simulink model "benign"  (R2017a)
settings: Solver=FixedStepDiscrete  StartTime=0.0  StopTime=100  FixedStep=1  RelTol=1e-3
model workspace (MAT data in the model file):
  ContractValidatorBlocksMap = containers.Map
  ContractValidatorBlocksMap.serialization.keys = {'benign/con_uas/validator', 'benign/contract/validator'}
  ContractValidatorBlocksMap.serialization.values{1}.block = 'benign/con_uas/validator'
  ContractValidatorBlocksMap.serialization.values{1}.assumePorts = 0
  ContractValidatorBlocksMap.serialization.values{1}.guaranteePorts = 8
  ContractValidatorBlocksMap.serialization.values{1}.modeBlocksPorts = 0
  ContractValidatorBlocksMap.serialization.values{1}.portHandles.Inport = [5488.14013672 5489.13989258 5490.13989258 5491.13989258 5492.13989258 5493.13989258 5494.13989258 5495.13989258]
  ContractValidatorBlocksMap.serialization.values{1}.portHandles.Outport = 5496.13989258
  ContractValidatorBlocksMap.serialization.values{1}.portHandles.Enable = []
  ContractValidatorBlocksMap.serialization.values{1}.portHandles.Trigger = []
  ContractValidatorBlocksMap.serialization.values{1}.portHandles.State = []
  ContractValidatorBlocksMap.serialization.values{1}.portHandles.LConn = []
  ContractValidatorBlocksMap.serialization.values{1}.portHandles.RConn = []
  ContractValidatorBlocksMap.serialization.values{1}.portHandles.Ifaction = []
  ContractValidatorBlocksMap.serialization.values{1}.portHandles.Reset = []
  ContractValidatorBlocksMap.serialization.values{1}.portConnectivity(1).Type = '1'
  ContractValidatorBlocksMap.serialization.values{1}.portConnectivity(1).Position = [390 -490]
  ContractValidatorBlocksMap.serialization.values{1}.portConnectivity(1).SrcBlock = 98.0086669922
  ContractValidatorBlocksMap.serialization.values{1}.portConnectivity(1).SrcPort = 0
  ContractValidatorBlocksMap.serialization.values{1}.portConnectivity(1).DstBlock = []
  ContractValidatorBlocksMap.serialization.values{1}.portConnectivity(1).DstPort = []
  ContractValidatorBlocksMap.serialization.values{1}.portConnectivity(2).Type = '2'
  ContractValidatorBlocksMap.serialization.values{1}.portConnectivity(2).Position = [390 -275]
  ContractValidatorBlocksMap.serialization.values{1}.portConnectivity(2).SrcBlock = 126.00793457
  ContractValidatorBlocksMap.serialization.values{1}.portConnectivity(2).SrcPort = 0
  ContractValidatorBlocksMap.serialization.values{1}.portConnectivity(2).DstBlock = []
  ContractValidatorBlocksMap.serialization.values{1}.portConnectivity(2).DstPort = []
  ContractValidatorBlocksMap.serialization.values{1}.portConnectivity(3).Type = '3'
  ContractValidatorBlocksMap.serialization.values{1}.portConnectivity(3).Position = [390 -60]
  ContractValidatorBlocksMap.serialization.values{1}.portConnectivity(3).SrcBlock = 154.008300781
  ContractValidatorBlocksMap.serialization.values{1}.portConnectivity(3).SrcPort = 0
  ContractValidatorBlocksMap.serialization.values{1}.portConnectivity(3).DstBlock = []
  ContractValidatorBlocksMap.serialization.values{1}.portConnectivity(3).DstPort = []
  ContractValidatorBlocksMap.serialization.values{1}.portConnectivity(4).Type = '4'
  ContractValidatorBlocksMap.serialization.values{1}.portConnectivity(4).Position = [390 155]
  ContractValidatorBlocksMap.serialization.values{1}.portConnectivity(4).SrcBlock = 184.007324219
  ContractValidatorBlocksMap.serialization.values{1}.portConnectivity(4).SrcPort = 0
  ContractValidatorBlocksMap.serialization.values{1}.portConnectivity(4).DstBlock = []
  ContractValidatorBlocksMap.serialization.values{1}.portConnectivity(4).DstPort = []
  ContractValidatorBlocksMap.serialization.values{1}.portConnectivity(5).Type = '5'
  ContractValidatorBlocksMap.serialization.values{1}.portConnectivity(5).Position = [390 370]
  ContractValidatorBlocksMap.serialization.values{1}.portConnectivity(5).SrcBlock = 214.006591797
  ContractValidatorBlocksMap.serialization.values{1}.portConnectivity(5).SrcPort = 0
  ContractValidatorBlocksMap.serialization.values{1}.portConnectivity(5).DstBlock = []
  ContractValidatorBlocksMap.serialization.values{1}.portConnectivity(5).DstPort = []
  ContractValidatorBlocksMap.serialization.values{1}.portConnectivity(6).Type = '6'
  ContractValidatorBlocksMap.serialization.values{1}.portConnectivity(6).Position = [390 585]
  ContractValidatorBlocksMap.serialization.values{1}.portConnectivity(6).SrcBlock = 254.006347656
  ContractValidatorBlocksMap.serialization.values{1}.portConnectivity(6).SrcPort = 0
  ContractValidatorBlocksMap.serialization.values{1}.portConnectivity(6).DstBlock = []
  ContractValidatorBlocksMap.serialization.values{1}.portConnectivity(6).DstPort = []
  ContractValidatorBlocksMap.serialization.values{1}.portConnectivity(7).Type = '7'
  ContractValidatorBlocksMap.serialization.values{1}.portConnectivity(7).Position = [390 800]
  ContractValidatorBlocksMap.serialization.values{1}.portConnectivity(7).SrcBlock = 294.005859375
  ContractValidatorBlocksMap.serialization.values{1}.portConnectivity(7).SrcPort = 0
  ContractValidatorBlocksMap.serialization.values{1}.portConnectivity(7).DstBlock = []
  ContractValidatorBlocksMap.serialization.values{1}.portConnectivity(7).DstPort = []
  ContractValidatorBlocksMap.serialization.values{1}.portConnectivity(8).Type = '8'
  ContractValidatorBlocksMap.serialization.values{1}.portConnectivity(8).Position = [390 1015]
  ContractValidatorBlocksMap.serialization.values{1}.portConnectivity(8).SrcBlock = 334.007080078
  ContractValidatorBlocksMap.serialization.values{1}.portConnectivity(8).SrcPort = 0
  ContractValidatorBlocksMap.serialization.values{1}.portConnectivity(8).DstBlock = []
  ContractValidatorBlocksMap.serialization.values{1}.portConnectivity(8).DstPort = []
  ContractValidatorBlocksMap.serialization.values{1}.portConnectivity(9).Type = '1'
  ContractValidatorBlocksMap.serialization.values{1}.portConnectivity(9).Position = [615 265]
  ContractValidatorBlocksMap.serialization.values{1}.portConnectivity(9).SrcBlock = []
  ContractValidatorBlocksMap.serialization.values{1}.portConnectivity(9).SrcPort = []
  ContractValidatorBlocksMap.serialization.values{1}.portConnectivity(9).DstBlock = 376.00793457
  ContractValidatorBlocksMap.serialization.values{1}.portConnectivity(9).DstPort = 0
  ContractValidatorBlocksMap.serialization.values{2}.block = 'benign/contract/validator'
  ContractValidatorBlocksMap.serialization.values{2}.assumePorts = 1
  ContractValidatorBlocksMap.serialization.values{2}.guaranteePorts = 1
  ContractValidatorBlocksMap.serialization.values{2}.modeBlocksPorts = 3
  ContractValidatorBlocksMap.serialization.values{2}.portHandles.Inport = [15090.0004883 15091.0004883 14397.0036621 15089.0006104 14391.0037842]
  ContractValidatorBlocksMap.serialization.values{2}.portHandles.Outport = 5595.05529785
  ContractValidatorBlocksMap.serialization.values{2}.portHandles.Enable = []
  ContractValidatorBlocksMap.serialization.values{2}.portHandles.Trigger = []
  ContractValidatorBlocksMap.serialization.values{2}.portHandles.State = []
  ContractValidatorBlocksMap.serialization.values{2}.portHandles.LConn = []
  ContractValidatorBlocksMap.serialization.values{2}.portHandles.RConn = []
  ContractValidatorBlocksMap.serialization.values{2}.portHandles.Ifaction = []
  ContractValidatorBlocksMap.serialization.values{2}.portHandles.Reset = []
  ContractValidatorBlocksMap.serialization.values{2}.portConnectivity(1).Type = '1'
  ContractValidatorBlocksMap.serialization.values{2}.portConnectivity(1).Position = [365 -125]
  ContractValidatorBlocksMap.serialization.values{2}.portConnectivity(1).SrcBlock = 15175.0004883
  ContractValidatorBlocksMap.serialization.values{2}.portConnectivity(1).SrcPort = 0
  ContractValidatorBlocksMap.serialization.values{2}.portConnectivity(1).DstBlock = []
  ContractValidatorBlocksMap.serialization.values{2}.portConnectivity(1).DstPort = []
  ContractValidatorBlocksMap.serialization.values{2}.portConnectivity(2).Type = '2'
  ContractValidatorBlocksMap.serialization.values{2}.portConnectivity(2).Position = [365 -25]
  ContractValidatorBlocksMap.serialization.values{2}.portConnectivity(2).SrcBlock = 15178.0007324
  ContractValidatorBlocksMap.serialization.values{2}.portConnectivity(2).SrcPort = 0
  ContractValidatorBlocksMap.serialization.values{2}.portConnectivity(2).DstBlock = []
  ContractValidatorBlocksMap.serialization.values{2}.portConnectivity(2).DstPort = []
  ContractValidatorBlocksMap.serialization.values{2}.portConnectivity(3).Type = '3'
  ContractValidatorBlocksMap.serialization.values{2}.portConnectivity(3).Position = [365 75]
  ContractValidatorBlocksMap.serialization.values{2}.portConnectivity(3).SrcBlock = 15181.0007324
  ContractValidatorBlocksMap.serialization.values{2}.portConnectivity(3).SrcPort = 0
  ContractValidatorBlocksMap.serialization.values{2}.portConnectivity(3).DstBlock = []
  ContractValidatorBlocksMap.serialization.values{2}.portConnectivity(3).DstPort = []
  ContractValidatorBlocksMap.serialization.values{2}.portConnectivity(4).Type = '4'
  ContractValidatorBlocksMap.serialization.values{2}.portConnectivity(4).Position = [365 175]
  ContractValidatorBlocksMap.serialization.values{2}.portConnectivity(4).SrcBlock = 15204.0007324
  ContractValidatorBlocksMap.serialization.values{2}.portConnectivity(4).SrcPort = 0
  ContractValidatorBlocksMap.serialization.values{2}.portConnectivity(4).DstBlock = []
  ContractValidatorBlocksMap.serialization.values{2}.portConnectivity(4).DstPort = []
  ContractValidatorBlocksMap.serialization.values{2}.portConnectivity(5).Type = '5'
  ContractValidatorBlocksMap.serialization.values{2}.portConnectivity(5).Position = [365 275]
  ContractValidatorBlocksMap.serialization.values{2}.portConnectivity(5).SrcBlock = 15227.0007324
  ContractValidatorBlocksMap.serialization.values{2}.portConnectivity(5).SrcPort = 0
  ContractValidatorBlocksMap.serialization.values{2}.portConnectivity(5).DstBlock = []
  ContractValidatorBlocksMap.serialization.values{2}.portConnectivity(5).DstPort = []
  ContractValidatorBlocksMap.serialization.values{2}.portConnectivity(6).Type = '1'
  ContractValidatorBlocksMap.serialization.values{2}.portConnectivity(6).Position = [500 75]
  ContractValidatorBlocksMap.serialization.values{2}.portConnectivity(6).SrcBlock = []
  ContractValidatorBlocksMap.serialization.values{2}.portConnectivity(6).SrcPort = []
  ContractValidatorBlocksMap.serialization.values{2}.portConnectivity(6).DstBlock = 5588.05688477
  ContractValidatorBlocksMap.serialization.values{2}.portConnectivity(6).DstPort = 0
  ContractValidatorBlocksMap.serialization.uniformity = 0
  ContractValidatorBlocksMap.serialization.keyType = 'char'
  ContractValidatorBlocksMap.serialization.valueType = 'any'
undefined symbols (not defined in the file or in its folder): contractAfterSimulation, contractBeforeSimulation, saveValidatorParameters
undefined symbols (not defined in the file): ContractBlock, ContractGuaranteeBlock, ContractValidatorBlock
libraries: simulink x436, CoCoSimSpecification x31
(part 1 of 3)
settings Model: Creator=mudat  LastModifiedBy=mudat

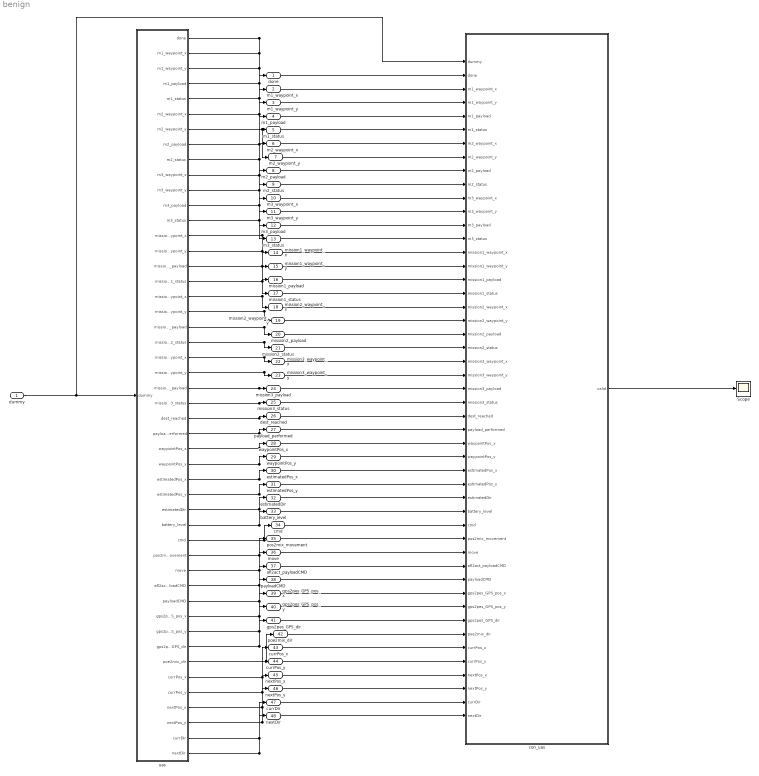
== system benign ==
  dummy : Inport  OutDataTypeStr=boolean
  Scope : Scope
  con_uas : Subsystem  mask(ContractBlock){ContractBlockType=ContractBlock}
      mask init:
      | set_param(gcb, 'LinkStatus', 'none');
      settings: CopyFcn=set_param(gcb, 'LinkStatus', 'none');
      mask DialogControl DescTextVar Prompt: Contract block
      mask Display:
      | text(0.5, 0.5, '{\bf\fontsize{20}Contract}', 'hor', 'center', 'texmode','on');
      | blocks = find_system(gcb, 'LookUnderMasks','all', 'SearchDepth',1,'BlockType','Inport');
      | for i = 1 : length(blocks)
      |     blockName = get_param(blocks(i), 'Name');
      |     [path, blockName] = fileparts(char(blockName));
      |     port_label('input', i, blockName);
      | end
      | 
      | blocks = find_system(gcb, 'LookUnderMasks','all', 'SearchDepth',1,'BlockType','Outport');
      | for i = 1 : length(blocks)
      |     blockName = get_param(blocks(i), 'Name');
      |     [path, blockName] = fileparts(char(blockName));
      |     port_label('output', i, blockName);
      | end
  uas : Subsystem
  done : Outport  OutDataTypeStr=boolean
  m1_waypoint_x : Outport  Port=2  OutDataTypeStr=int32
  m1_waypoint_y : Outport  Port=3  OutDataTypeStr=int32
  m1_payload : Outport  Port=4  OutDataTypeStr=int32
  m1_status : Outport  Port=5  OutDataTypeStr=int32
  m2_waypoint_x : Outport  Port=6  OutDataTypeStr=int32
  m2_waypoint_y : Outport  Port=7  OutDataTypeStr=int32
  m2_payload : Outport  Port=8  OutDataTypeStr=int32
  m2_status : Outport  Port=9  OutDataTypeStr=int32
  m3_waypoint_x : Outport  Port=10  OutDataTypeStr=int32
  m3_waypoint_y : Outport  Port=11  OutDataTypeStr=int32
  m3_payload : Outport  Port=12  OutDataTypeStr=int32
  m3_status : Outport  Port=13  OutDataTypeStr=int32
  mission1_waypoint_x : Outport  Port=14  OutDataTypeStr=int32
  mission1_waypoint_y : Outport  Port=15  OutDataTypeStr=int32
  mission1_payload : Outport  Port=16  OutDataTypeStr=int32
  mission1_status : Outport  Port=17  OutDataTypeStr=int32
  mission2_waypoint_x : Outport  Port=18  OutDataTypeStr=int32
  mission2_waypoint_y : Outport  Port=19  OutDataTypeStr=int32
  mission2_payload : Outport  Port=20  OutDataTypeStr=int32
  mission2_status : Outport  Port=21  OutDataTypeStr=int32
  mission3_waypoint_x : Outport  Port=22  OutDataTypeStr=int32
  mission3_waypoint_y : Outport  Port=23  OutDataTypeStr=int32
  mission3_payload : Outport  Port=24  OutDataTypeStr=int32
  mission3_status : Outport  Port=25  OutDataTypeStr=int32
  dest_reached : Outport  Port=26  OutDataTypeStr=boolean
  payload_performed : Outport  Port=27  OutDataTypeStr=boolean
  waypointPos_x : Outport  Port=28  OutDataTypeStr=int32
  waypointPos_y : Outport  Port=29  OutDataTypeStr=int32
  estimatedPos_x : Outport  Port=30  OutDataTypeStr=int32
  estimatedPos_y : Outport  Port=31  OutDataTypeStr=int32
  estimatedDir : Outport  Port=32  OutDataTypeStr=int32
  battery_level : Outport  Port=33  OutDataTypeStr=int32
  cmd : Outport  Port=34  OutDataTypeStr=int32
  pos2mix_movement : Outport  Port=35  OutDataTypeStr=int32
  move : Outport  Port=36  OutDataTypeStr=int32
  afl2act_payloadCMD : Outport  Port=37  OutDataTypeStr=int32
  payloadCMD : Outport  Port=38  OutDataTypeStr=int32
  gps2pes_GPS_pos_x : Outport  Port=39  OutDataTypeStr=int32
  gps2pes_GPS_pos_y : Outport  Port=40  OutDataTypeStr=int32
  gps2pes_GPS_dir : Outport  Port=41  OutDataTypeStr=int32
  poe2mix_dir : Outport  Port=42  OutDataTypeStr=int32
  currPos_x : Outport  Port=43  OutDataTypeStr=int32
  currPos_y : Outport  Port=44  OutDataTypeStr=int32
  nextPos_x : Outport  Port=45  OutDataTypeStr=int32
  nextPos_y : Outport  Port=46  OutDataTypeStr=int32
  currDir : Outport  Port=47  OutDataTypeStr=int32
  nextDir : Outport  Port=48  OutDataTypeStr=int32
  wires:
  dummy/1 -> con_uas/1(dummy), uas/1(dummy)
  uas/1(done) -> done/1, con_uas/2(done)
  uas/2(m1_waypoint_x) -> m1_waypoint_x/1, con_uas/3(m1_waypoint_x)
  uas/3(m1_waypoint_y) -> m1_waypoint_y/1, con_uas/4(m1_waypoint_y)
  uas/4(m1_payload) -> m1_payload/1, con_uas/5(m1_payload)
  uas/5(m1_status) -> m1_status/1, con_uas/6(m1_status)
  uas/6(m2_waypoint_x) -> m2_waypoint_x/1, con_uas/7(m2_waypoint_x)
  uas/7(m2_waypoint_y) -> m2_waypoint_y/1, con_uas/8(m2_waypoint_y)
  uas/8(m2_payload) -> m2_payload/1, con_uas/9(m2_payload)
  uas/9(m2_status) -> m2_status/1, con_uas/10(m2_status)
  uas/10(m3_waypoint_x) -> m3_waypoint_x/1, con_uas/11(m3_waypoint_x)
  uas/11(m3_waypoint_y) -> m3_waypoint_y/1, con_uas/12(m3_waypoint_y)
  uas/12(m3_payload) -> m3_payload/1, con_uas/13(m3_payload)
  uas/13(m3_status) -> m3_status/1, con_uas/14(m3_status)
  uas/14(mission1_waypoint_x) -> mission1_waypoint_x/1, con_uas/15(mission1_waypoint_x)
  uas/15(mission1_waypoint_y) -> mission1_waypoint_y/1, con_uas/16(mission1_waypoint_y)
  uas/16(mission1_payload) -> mission1_payload/1, con_uas/17(mission1_payload)
  uas/17(mission1_status) -> mission1_status/1, con_uas/18(mission1_status)
  uas/18(mission2_waypoint_x) -> mission2_waypoint_x/1, con_uas/19(mission2_waypoint_x)
  uas/19(mission2_waypoint_y) -> mission2_waypoint_y/1, con_uas/20(mission2_waypoint_y)
  uas/20(mission2_payload) -> mission2_payload/1, con_uas/21(mission2_payload)
  uas/21(mission2_status) -> mission2_status/1, con_uas/22(mission2_status)
  uas/22(mission3_waypoint_x) -> mission3_waypoint_x/1, con_uas/23(mission3_waypoint_x)
  uas/23(mission3_waypoint_y) -> mission3_waypoint_y/1, con_uas/24(mission3_waypoint_y)
  uas/24(mission3_payload) -> mission3_payload/1, con_uas/25(mission3_payload)
  uas/25(mission3_status) -> mission3_status/1, con_uas/26(mission3_status)
  uas/26(dest_reached) -> dest_reached/1, con_uas/27(dest_reached)
  uas/27(payload_performed) -> payload_performed/1, con_uas/28(payload_performed)
  uas/28(waypointPos_x) -> waypointPos_x/1, con_uas/29(waypointPos_x)
  uas/29(waypointPos_y) -> waypointPos_y/1, con_uas/30(waypointPos_y)
  uas/30(estimatedPos_x) -> estimatedPos_x/1, con_uas/31(estimatedPos_x)
  uas/31(estimatedPos_y) -> estimatedPos_y/1, con_uas/32(estimatedPos_y)
  uas/32(estimatedDir) -> estimatedDir/1, con_uas/33(estimatedDir)
  uas/33(battery_level) -> battery_level/1, con_uas/34(battery_level)
  uas/34(cmd) -> cmd/1, con_uas/35(cmd)
  uas/35(pos2mix_movement) -> pos2mix_movement/1, con_uas/36(pos2mix_movement)
  uas/36(move) -> move/1, con_uas/37(move)
  uas/37(afl2act_payloadCMD) -> afl2act_payloadCMD/1, con_uas/38(afl2act_payloadCMD)
  uas/38(payloadCMD) -> payloadCMD/1, con_uas/39(payloadCMD)
  uas/39(gps2pes_GPS_pos_x) -> gps2pes_GPS_pos_x/1, con_uas/40(gps2pes_GPS_pos_x)
  uas/40(gps2pes_GPS_pos_y) -> gps2pes_GPS_pos_y/1, con_uas/41(gps2pes_GPS_pos_y)
  uas/41(gps2pes_GPS_dir) -> gps2pes_GPS_dir/1, con_uas/42(gps2pes_GPS_dir)
  uas/42(poe2mix_dir) -> poe2mix_dir/1, con_uas/43(poe2mix_dir)
  uas/43(currPos_x) -> currPos_x/1, con_uas/44(currPos_x)
  uas/44(currPos_y) -> currPos_y/1, con_uas/45(currPos_y)
  uas/45(nextPos_x) -> nextPos_x/1, con_uas/46(nextPos_x)
  uas/46(nextPos_y) -> nextPos_y/1, con_uas/47(nextPos_y)
  uas/47(currDir) -> currDir/1, con_uas/48(currDir)
  uas/48(nextDir) -> nextDir/1, con_uas/49(nextDir)
  con_uas/1(valid) -> Scope/1

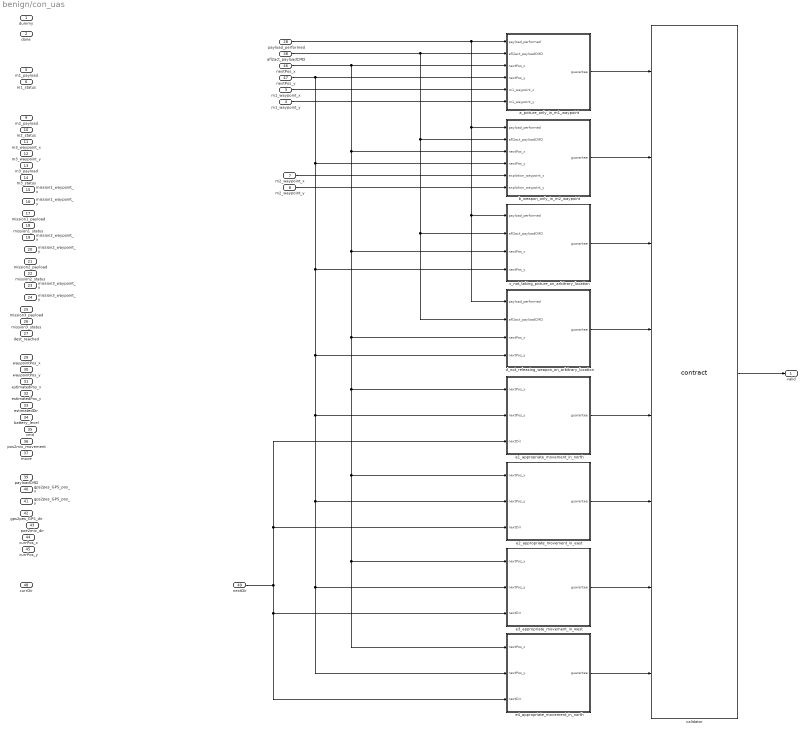
== system benign/con_uas ==
  dummy : Inport
  done : Inport  Port=2
  m1_waypoint_x : Inport  Port=3
  m1_waypoint_y : Inport  Port=4
  m1_payload : Inport  Port=5
  m1_status : Inport  Port=6
  m2_waypoint_x : Inport  Port=7
  m2_waypoint_y : Inport  Port=8
  m2_payload : Inport  Port=9
  m2_status : Inport  Port=10
  m3_waypoint_x : Inport  Port=11
  m3_waypoint_y : Inport  Port=12
  m3_payload : Inport  Port=13
  m3_status : Inport  Port=14
  mission1_waypoint_x : Inport  Port=15
  mission1_waypoint_y : Inport  Port=16
  mission1_payload : Inport  Port=17
  mission1_status : Inport  Port=18
  mission2_waypoint_x : Inport  Port=19
  mission2_waypoint_y : Inport  Port=20
  mission2_payload : Inport  Port=21
  mission2_status : Inport  Port=22
  mission3_waypoint_x : Inport  Port=23
  mission3_waypoint_y : Inport  Port=24
  mission3_payload : Inport  Port=25
  mission3_status : Inport  Port=26
  dest_reached : Inport  Port=27
  payload_performed : Inport  Port=28
  waypointPos_x : Inport  Port=29
  waypointPos_y : Inport  Port=30
  estimatedPos_x : Inport  Port=31
  estimatedPos_y : Inport  Port=32
  estimatedDir : Inport  Port=33
  battery_level : Inport  Port=34
  cmd : Inport  Port=35
  pos2mix_movement : Inport  Port=36
  move : Inport  Port=37
  afl2act_payloadCMD : Inport  Port=38
  payloadCMD : Inport  Port=39
  gps2pes_GPS_pos_x : Inport  Port=40
  gps2pes_GPS_pos_y : Inport  Port=41
  gps2pes_GPS_dir : Inport  Port=42
  poe2mix_dir : Inport  Port=43
  currPos_x : Inport  Port=44
  currPos_y : Inport  Port=45
  nextPos_x : Inport  Port=46
  nextPos_y : Inport  Port=47
  currDir : Inport  Port=48
  nextDir : Inport  Port=49
  a_picture_only_in_m1_waypoint : Subsystem  mask(ContractGuaranteeBlock){ContractBlockType=ContractGuaranteeBlock}
      mask init:
      | set_param(gcb, 'LinkStatus', 'none');
      mask DialogControl DescTextVar Prompt: Guarantee block
  b_weapon_only_in_m2_waypoint : Subsystem  mask(ContractGuaranteeBlock){ContractBlockType=ContractGuaranteeBlock}
      mask init:
      | set_param(gcb, 'LinkStatus', 'none');
      mask DialogControl DescTextVar Prompt: Guarantee block
  c_not_taking_picture_on_arbitrary_location : Subsystem  mask(ContractGuaranteeBlock){ContractBlockType=ContractGuaranteeBlock}
      mask init:
      | set_param(gcb, 'LinkStatus', 'none');
      mask DialogControl DescTextVar Prompt: Guarantee block
  d_not_releasing_weapon_on_arbitrary_location : Subsystem  mask(ContractGuaranteeBlock){ContractBlockType=ContractGuaranteeBlock}
      mask init:
      | set_param(gcb, 'LinkStatus', 'none');
      mask DialogControl DescTextVar Prompt: Guarantee block
  e1_appropriate_movement_in_north : Subsystem  mask(ContractGuaranteeBlock){ContractBlockType=ContractGuaranteeBlock}
      mask init:
      | set_param(gcb, 'LinkStatus', 'none');
      mask DialogControl DescTextVar Prompt: Guarantee block
  e2_appropriate_movement_in_east : Subsystem  mask(ContractGuaranteeBlock){ContractBlockType=ContractGuaranteeBlock}
      mask init:
      | set_param(gcb, 'LinkStatus', 'none');
      mask DialogControl DescTextVar Prompt: Guarantee block
  e3_appropriate_movement_in_west : Subsystem  mask(ContractGuaranteeBlock){ContractBlockType=ContractGuaranteeBlock}
      mask init:
      | set_param(gcb, 'LinkStatus', 'none');
      mask DialogControl DescTextVar Prompt: Guarantee block
  e4_appropriate_movement_in_north : Subsystem  mask(ContractGuaranteeBlock){ContractBlockType=ContractGuaranteeBlock}
      mask init:
      | set_param(gcb, 'LinkStatus', 'none');
      mask DialogControl DescTextVar Prompt: Guarantee block
  validator : M-S-Function  LoadFcn=saveValidatorParameters(gcb);  InitFcn=contractBeforeSimulation();  StopFcn=contractAfterSimulation();  FunctionName=contract  mask(ContractValidatorBlock){assumePorts=0, guaranteePorts=8, modePorts=0, ContractBlockType=ContractValidatorBlock, createInportsCheckbox=off}
      mask prompts: assumePorts "Assume ports     :"; guaranteePorts "Guarantee ports :"; modePorts "Mode ports        :"; createInportsCheckbox "Create inports and connect them automatically"
      mask init:
      | set_param(gcb,'LinkStatus','none');
      | contract_callback('inputs_callback',gcb);
      mask DialogControl DescTextVar Prompt: The validator block implements the following logic: <br> <br> <b>Sofar</b>(assume<sub>1</sub> <b>&#8743;</b> assume<sub>2</sub> <b>&#8743;</b> ... assume<sub>k</sub>) <b>&rarr;</b> (guarantee<sub>1</sub> <b>&#8743;</b> guarantee<sub>2</sub> <b>&#8743;</b> ... guarantee<sub>m</sub> <b>&#8743;</b>  mode<sub>1</sub> <b>&#8743;</b> mode<sub>2</sub> <b>&#8743;</b> ... <b>&#8743;</b> mode<sub>n</sub> )<br> where mode<sub>i</sub> = require<sub>i</sub> <b>&rarr;</b> ensure<sub>i</sub>
      mask Display:
      | color('black');
      | port_label('input',1,'guarantee');
      | port_label('input',2,'guarantee');
      | port_label('input',3,'guarantee');
      | port_label('input',4,'guarantee');
      | port_label('input',5,'guarantee');
      | port_label('input',6,'guarantee');
      | port_label('input',7,'guarantee');
      | port_label('input',8,'guarantee');
      | port_label('output',1,'valid');
  valid : Outport
  wires:
  validator/1 -> valid/1
  m1_waypoint_x/1 -> a_picture_only_in_m1_waypoint/5(m1_waypoint_x)
  m1_waypoint_y/1 -> a_picture_only_in_m1_waypoint/6(m1_waypoint_y)
  m2_waypoint_x/1 -> b_weapon_only_in_m2_waypoint/5(explotion_waypoint_x)
  m2_waypoint_y/1 -> b_weapon_only_in_m2_waypoint/6(explotion_waypoint_y)
  payload_performed/1 -> d_not_releasing_weapon_on_arbitrary_location/1(payload_performed), c_not_taking_picture_on_arbitrary_location/1(payload_performed), b_weapon_only_in_m2_waypoint/1(payload_performed), a_picture_only_in_m1_waypoint/1(payload_performed)
  afl2act_payloadCMD/1 -> d_not_releasing_weapon_on_arbitrary_location/2(afl2act_payloadCMD), c_not_taking_picture_on_arbitrary_location/2(afl2act_payloadCMD), b_weapon_only_in_m2_waypoint/2(afl2act_payloadCMD), a_picture_only_in_m1_waypoint/2(afl2act_payloadCMD)
  nextDir/1 -> e3_appropriate_movement_in_west/3(nextDir), e4_appropriate_movement_in_north/3(nextDir), e2_appropriate_movement_in_east/3(nextDir), e1_appropriate_movement_in_north/3(nextDir)
  a_picture_only_in_m1_waypoint/1(guarantee) -> validator/1
  b_weapon_only_in_m2_waypoint/1(guarantee) -> validator/2
  c_not_taking_picture_on_arbitrary_location/1(guarantee) -> validator/3
  d_not_releasing_weapon_on_arbitrary_location/1(guarantee) -> validator/4
  e1_appropriate_movement_in_north/1(guarantee) -> validator/5
  e2_appropriate_movement_in_east/1(guarantee) -> validator/6
  e3_appropriate_movement_in_west/1(guarantee) -> validator/7
  nextPos_x/1 -> e4_appropriate_movement_in_north/1(nextPos_x), e3_appropriate_movement_in_west/1(nextPos_x), e2_appropriate_movement_in_east/1(nextPos_x), e1_appropriate_movement_in_north/1(nextPos_x), d_not_releasing_weapon_on_arbitrary_location/3(nextPos_x), c_not_taking_picture_on_arbitrary_location/3(nextPos_x), b_weapon_only_in_m2_waypoint/3(nextPos_x), a_picture_only_in_m1_waypoint/3(nextPos_x)
  nextPos_y/1 -> e4_appropriate_movement_in_north/2(nextPos_y), e3_appropriate_movement_in_west/2(nextPos_y), e2_appropriate_movement_in_east/2(nextPos_y), e1_appropriate_movement_in_north/2(nextPos_y), d_not_releasing_weapon_on_arbitrary_location/4(nextPos_y), c_not_taking_picture_on_arbitrary_location/4(nextPos_y), b_weapon_only_in_m2_waypoint/4(nextPos_y), a_picture_only_in_m1_waypoint/4(nextPos_y)
  e4_appropriate_movement_in_north/1(guarantee) -> validator/8

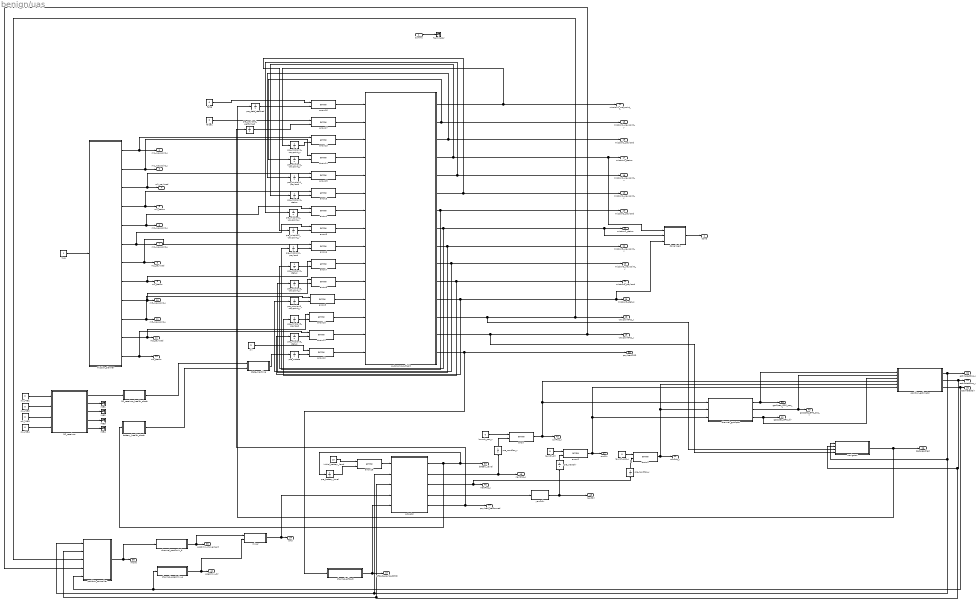
== system benign/uas ==
  dummy : Inport  OutDataTypeStr=boolean
  MIE{1..4} (4 alike) : Terminator
  RC_receiver : Subsystem
  RC_receiver_health_check : Subsystem
  Terminator : Terminator
  actuator : Subsystem
  arrow{,1..18} (19 alike) : CoCoSimSpecification/arrow  LustreOperatorBlock=ArrowOperator
      settings: SourceProductName=CoCoSim Specification
  autonomous_flight : Subsystem
  battery_health_check : Subsystem
  channel_afl2act : Subsystem
  channel_gps2pes : Subsystem
  channel_poe2mix_a : Subsystem
  channel_poe2mix_b : Subsystem
  done logic : Subsystem
  false : Constant  Value=0  OutDataTypeStr=boolean
  false1 : Constant  Value=0  OutDataTypeStr=boolean
  initial_battery_level : Constant  Value=15  OutDataTypeStr=int32
  launch_dir : Constant  Value=0  OutDataTypeStr=int32
  launch_pos_x : Constant  Value=0  OutDataTypeStr=int32
  launch_pos_y : Constant  Value=0  OutDataTypeStr=int32
  mission_planner : Subsystem
  mixer : Subsystem
  navigator : Subsystem
  position_controller : Subsystem
  position_estimator : Subsystem
  pre_battery_level : UnitDelay  SampleTime=-1
  pre_dest_reached : UnitDelay  SampleTime=-1
  pre_mission1_payload : UnitDelay  SampleTime=-1
  pre_mission1_status : UnitDelay  SampleTime=-1
  pre_mission1_waypoint_x : UnitDelay  SampleTime=-1
  pre_mission1_waypoint_y : UnitDelay  SampleTime=-1
  pre_mission2_payload : UnitDelay  SampleTime=-1
  pre_mission2_status : UnitDelay  SampleTime=-1
  pre_mission2_waypoint_x : UnitDelay  SampleTime=-1
  pre_mission2_waypoint_y : UnitDelay  SampleTime=-1
  pre_mission3_payload : UnitDelay  SampleTime=-1
  pre_mission3_status : UnitDelay  SampleTime=-1
  pre_mission3_waypoint_x : UnitDelay  SampleTime=-1
  pre_mission3_waypoint_y : UnitDelay  SampleTime=-1
  pre_mstate : UnitDelay  SampleTime=-1
  pre_nextDir : UnitDelay  SampleTime=-1
  pre_nextPos_x : UnitDelay  SampleTime=-1
  pre_nextPos_y : UnitDelay  SampleTime=-1
  pre_payload_performed : UnitDelay  SampleTime=-1
  rcv_MIE{1..4} (4 alike) : Constant  Value=0  OutDataTypeStr=int32
  six : Constant  Value=6  OutDataTypeStr=int32
  state_machine : Subsystem
  true : Constant  OutDataTypeStr=boolean
  yaw2dir : Subsystem
  done : Outport  OutDataTypeStr=boolean
  m1_waypoint_x : Outport  Port=2  OutDataTypeStr=int32
  m1_waypoint_y : Outport  Port=3  OutDataTypeStr=int32
  m1_payload : Outport  Port=4  OutDataTypeStr=int32
  m1_status : Outport  Port=5  OutDataTypeStr=int32
  m2_waypoint_x : Outport  Port=6  OutDataTypeStr=int32
  m2_waypoint_y : Outport  Port=7  OutDataTypeStr=int32
  m2_payload : Outport  Port=8  OutDataTypeStr=int32
  m2_status : Outport  Port=9  OutDataTypeStr=int32
  m3_waypoint_x : Outport  Port=10  OutDataTypeStr=int32
  m3_waypoint_y : Outport  Port=11  OutDataTypeStr=int32
  m3_payload : Outport  Port=12  OutDataTypeStr=int32
  m3_status : Outport  Port=13  OutDataTypeStr=int32
  mission1_waypoint_x : Outport  Port=14  OutDataTypeStr=int32
  mission1_waypoint_y : Outport  Port=15  OutDataTypeStr=int32
  mission1_payload : Outport  Port=16  OutDataTypeStr=int32
  mission1_status : Outport  Port=17  OutDataTypeStr=int32
  mission2_waypoint_x : Outport  Port=18  OutDataTypeStr=int32
  mission2_waypoint_y : Outport  Port=19  OutDataTypeStr=int32
  mission2_payload : Outport  Port=20  OutDataTypeStr=int32
  mission2_status : Outport  Port=21  OutDataTypeStr=int32
  mission3_waypoint_x : Outport  Port=22  OutDataTypeStr=int32
  mission3_waypoint_y : Outport  Port=23  OutDataTypeStr=int32
  mission3_payload : Outport  Port=24  OutDataTypeStr=int32
  mission3_status : Outport  Port=25  OutDataTypeStr=int32
  dest_reached : Outport  Port=26  OutDataTypeStr=boolean
  payload_performed : Outport  Port=27  OutDataTypeStr=boolean
  waypointPos_x : Outport  Port=28  OutDataTypeStr=int32
  waypointPos_y : Outport  Port=29  OutDataTypeStr=int32
  estimatedPos_x : Outport  Port=30  OutDataTypeStr=int32
  estimatedPos_y : Outport  Port=31  OutDataTypeStr=int32
  estimatedDir : Outport  Port=32  OutDataTypeStr=int32
  battery_level : Outport  Port=33  OutDataTypeStr=int32
  cmd : Outport  Port=34  OutDataTypeStr=int32
  pos2mix_movement : Outport  Port=35  OutDataTypeStr=int32
  move : Outport  Port=36  OutDataTypeStr=int32
  afl2act_payloadCMD : Outport  Port=37  OutDataTypeStr=int32
  payloadCMD : Outport  Port=38  OutDataTypeStr=int32
  gps2pes_GPS_pos_x : Outport  Port=39  OutDataTypeStr=int32
  gps2pes_GPS_pos_y : Outport  Port=40  OutDataTypeStr=int32
  gps2pes_GPS_dir : Outport  Port=41  OutDataTypeStr=int32
  poe2mix_dir : Outport  Port=42  OutDataTypeStr=int32
  currPos_x : Outport  Port=43  OutDataTypeStr=int32
  currPos_y : Outport  Port=44  OutDataTypeStr=int32
  nextPos_x : Outport  Port=45  OutDataTypeStr=int32
  nextPos_y : Outport  Port=46  OutDataTypeStr=int32
  currDir : Outport  Port=47  OutDataTypeStr=int32
  nextDir : Outport  Port=48  OutDataTypeStr=int32
  wires:
  true/1 -> mission_planner/1(dummy)
  mission_planner/1(m1_waypoint_x) -> arrow13/1, m1_waypoint_x/1
  mission_planner/2(m1_waypoint_y) -> arrow14/1, m1_waypoint_y/1
  mission_planner/3(m1_payload) -> arrow15/1, m1_payload/1
  mission_planner/4(m1_status) -> arrow3/1, m1_status/1
  mission_planner/5(m2_waypoint_x) -> arrow4/1, m2_waypoint_x/1
  mission_planner/6(m2_waypoint_y) -> m2_waypoint_y/1, arrow5/1
  mission_planner/7(m2_payload) -> arrow6/1, m2_payload/1
  mission_planner/8(m2_status) -> arrow7/1, m2_status/1
  mission_planner/9(m3_waypoint_x) -> arrow8/1, m3_waypoint_x/1
  mission_planner/10(m3_waypoint_y) -> arrow9/1, m3_waypoint_y/1
  mission_planner/11(m3_payload) -> arrow10/1, m3_payload/1
  mission_planner/12(m3_status) -> arrow11/1, m3_status/1
  launch_pos_x/1 -> arrow/1
  arrow/1 -> currPos_x/1, position_estimator/4(currPos_x), channel_gps2pes/1(currPos_x)
  launch_pos_y/1 -> arrow1/1
  arrow1/1 -> currPos_y/1, position_estimator/5(currPos_y), channel_gps2pes/2(currPos_y)
  actuator/1(new_battery_level) -> battery_health_check/1(battery_level), pre_battery_level/1, battery_level/1
  actuator/2(nextPos_x) -> nextPos_x/1, pre_nextPos_x/1
  actuator/3(nextPos_y) -> pre_nextPos_y/1, nextPos_y/1
  actuator/5(payload_performed) -> pre_payload_performed/1, payload_performed/1
  arrow2/1 -> channel_gps2pes/3(currDir), position_estimator/6(currDir), currDir/1
  launch_dir/1 -> arrow2/1
  actuator/4(yaw) -> yaw2dir/1(yaw)
  yaw2dir/1(dir) -> nextDir/1, pre_nextDir/1
  channel_gps2pes/1(gps2pes_GPS_pos_x) -> gps2pes_GPS_pos_x/1, position_estimator/1(gps2pes_GPS_pos_x)
  channel_gps2pes/2(gps2pes_GPS_pos_y) -> gps2pes_GPS_pos_y/1, position_estimator/2(gps2pes_GPS_pos_y)
  channel_gps2pes/3(gps2pes_GPS_dir) -> position_estimator/3(gps2pes_GPS_dir), gps2pes_GPS_dir/1
  position_estimator/1(estimatedPos_x) -> navigator/1(estimatedPos_x), position_controller/1(currentPos_x), actuator/2(currentPos_x), estimatedPos_x/1
  position_estimator/2(estimatedPos_y) -> position_controller/2(currentPos_y), actuator/3(currentPos_y), navigator/2(estimatedPos_y), estimatedPos_y/1
  position_estimator/3(estimatedDir) -> position_controller/5(currentDir), channel_poe2mix_a/1(in_dir), estimatedDir/1
  autonomous_flight/1(upd_mission1_waypoint_x) -> pre_mission1_waypoint_x/1, mission1_waypoint_x/1
  autonomous_flight/2(upd_mission1_waypoint_y) -> mission1_waypoint_y/1, pre_mission1_waypoint_y/1
  autonomous_flight/3(upd_mission1_payload) -> mission1_payload/1, pre_mission1_payload/1
  autonomous_flight/4(upd_mission1_status) -> done logic/1(mission1_status), mission1_status/1, pre_mission1_status/1
  autonomous_flight/5(upd_mission2_waypoint_x) -> mission2_waypoint_x/1, pre_mission2_waypoint_x/1
  autonomous_flight/6(upd_mission2_waypoint_y) -> pre_mission2_waypoint_y/1, mission2_waypoint_y/1
  autonomous_flight/7(upd_mission2_payload) -> mission2_payload/1, pre_mission2_payload/1
  autonomous_flight/8(upd_mission2_status) -> pre_mission2_status/1, done logic/2(mission2_status), mission2_status/1
  autonomous_flight/9(upd_mission3_waypoint_x) -> pre_mission3_waypoint_x/1, mission3_waypoint_x/1
  autonomous_flight/10(upd_mission3_waypoint_y) -> pre_mission3_waypoint_y/1, mission3_waypoint_y/1
  autonomous_flight/11(upd_mission3_payload) -> pre_mission3_payload/1, mission3_payload/1
  autonomous_flight/12(upd_mission3_status) -> pre_mission3_status/1, done logic/3(mission3_status), mission3_status/1
  autonomous_flight/13(waypointPos_x) -> navigator/3(waypointPos_x), position_controller/3(waypointPos_x), waypointPos_x/1
  autonomous_flight/14(waypointPos_y) -> position_controller/4(waypointPos_y), waypointPos_y/1, navigator/4(waypointPos_y)
  autonomous_flight/15(payloadCMD) -> channel_afl2act/1(in_payloadCMD), payloadCMD/1
  false/1 -> arrow16/1
  false1/1 -> arrow17/1
  navigator/1(dest_reached) -> pre_dest_reached/1, dest_reached/1
  arrow16/1 -> autonomous_flight/1(dest_reached)
  arrow17/1 -> autonomous_flight/2(payload_performed)
  pre_payload_performed/1 -> arrow17/2
  pre_dest_reached/1 -> arrow16/2
  pre_nextPos_y/1 -> arrow1/2
  pre_nextPos_x/1 -> arrow/2
  pre_nextDir/1 -> arrow2/2
  arrow13/1 -> autonomous_flight/3(mission1_waypoint_x)
  arrow12/1 -> autonomous_flight/15(mstate)
  arrow11/1 -> autonomous_flight/14(mission3_status)
  arrow10/1 -> autonomous_flight/13(mission3_payload)
  arrow9/1 -> autonomous_flight/12(mission3_waypoint_y)
  arrow8/1 -> autonomous_flight/11(mission3_waypoint_x)
  arrow7/1 -> autonomous_flight/10(mission2_status)
  arrow6/1 -> autonomous_flight/9(mission2_payload)
  arrow5/1 -> autonomous_flight/8(mission2_waypoint_y)
  arrow4/1 -> autonomous_flight/7(mission2_waypoint_x)
  arrow3/1 -> autonomous_flight/6(mission1_status)
  arrow15/1 -> autonomous_flight/5(mission1_payload)
  arrow14/1 -> autonomous_flight/4(mission1_waypoint_y)
  pre_mission1_waypoint_x/1 -> arrow13/2
  pre_mission1_waypoint_y/1 -> arrow14/2
  pre_mission1_status/1 -> arrow3/2
  pre_mission1_payload/1 -> arrow15/2
  pre_mission2_waypoint_x/1 -> arrow4/2
  pre_mission2_waypoint_y/1 -> arrow5/2
  pre_mission2_payload/1 -> arrow6/2
  pre_mission2_status/1 -> arrow7/2
  pre_mission3_waypoint_x/1 -> arrow8/2
  pre_mission3_waypoint_y/1 -> arrow9/2
  pre_mission3_payload/1 -> arrow10/2
  pre_mission3_status/1 -> arrow11/2
  pre_mstate/1 -> arrow12/2
  state_machine/1(mstate) -> pre_mstate/1
  six/1 -> arrow12/1
  done logic/1(done) -> done/1
  RC_receiver_health_check/1(ATE6) -> state_machine/1(ATE6)
  RC_receiver/1(normal) -> RC_receiver_health_check/1(normal)
  battery_health_check/1(ATE7) -> state_machine/2(ATE7)
  rcv_MIE1/1 -> RC_receiver/1(rcv_MIE1)
  rcv_MIE2/1 -> RC_receiver/2(rcv_MIE2)
  rcv_MIE3/1 -> RC_receiver/3(rcv_MIE3)
  rcv_MIE4/1 -> RC_receiver/4(rcv_MIE4)
  RC_receiver/2(MIE1) -> MIE1/1
  RC_receiver/5(MIE4) -> MIE4/1
  RC_receiver/4(MIE3) -> MIE3/1
  RC_receiver/3(MIE2) -> MIE2/1
  initial_battery_level/1 -> arrow18/1
  arrow18/1 -> actuator/1(battery_level)
  pre_battery_level/1 -> arrow18/2
  mixer/1(cmd) -> actuator/4(cmd), cmd/1
  channel_afl2act/1(out_payloadCMD) -> actuator/5(payloadCMD), afl2act_payloadCMD/1
  channel_poe2mix_a/1(out_dir) -> mixer/2(currentDir), poe2mix_dir/1
  channel_poe2mix_b/1(out_movement) -> mixer/1(move), pos2mix_movement/1
  position_controller/1(move) -> channel_poe2mix_b/1(in_movement), move/1
  dummy/1 -> Terminator/1

== system benign/con_uas/a_picture_only_in_m1_waypoint ==
  payload_performed : Inport  OutDataTypeStr=boolean
  afl2act_payloadCMD : Inport  Port=2  OutDataTypeStr=int32
  nextPos_x : Inport  Port=3  OutDataTypeStr=int32
  nextPos_y : Inport  Port=4  OutDataTypeStr=int32
  m1_waypoint_x : Inport  Port=5  OutDataTypeStr=int32
  m1_waypoint_y : Inport  Port=6  OutDataTypeStr=int32
  Compare To Constant : simulink/Logic and Bit Operations/Compare To Constant  relop===  const=0  OutDataTypeStr=boolean
  Logical Operator1 : Logic  Operator=NOT  IconShape=distinctive  AllPortsSameDT=off  OutDataTypeStr=boolean
  Relational Operator : RelationalOperator  Operator===  OutDataTypeStr=boolean  RndMeth=Simplest
  Relational Operator1 : RelationalOperator  Operator===  OutDataTypeStr=boolean  RndMeth=Simplest
  and : Logic  IconShape=distinctive  AllPortsSameDT=off  OutDataTypeStr=boolean
  and1 : Logic  IconShape=distinctive  AllPortsSameDT=off  OutDataTypeStr=boolean
  or : Logic  Operator=OR  IconShape=distinctive  AllPortsSameDT=off  OutDataTypeStr=boolean
  guarantee : Outport  OutDataTypeStr=boolean
  wires:
  payload_performed/1 -> and/1
  afl2act_payloadCMD/1 -> Compare To Constant/1
  Compare To Constant/1 -> and/2
  and/1 -> Logical Operator1/1
  Logical Operator1/1 -> or/1
  or/1 -> guarantee/1
  nextPos_x/1 -> Relational Operator/1
  m1_waypoint_x/1 -> Relational Operator/2
  nextPos_y/1 -> Relational Operator1/1
  m1_waypoint_y/1 -> Relational Operator1/2
  Relational Operator/1 -> and1/1
  Relational Operator1/1 -> and1/2
  and1/1 -> or/2

== system benign/con_uas/b_weapon_only_in_m2_waypoint ==
  payload_performed : Inport  OutDataTypeStr=boolean
  afl2act_payloadCMD : Inport  Port=2  OutDataTypeStr=int32
  nextPos_x : Inport  Port=3  OutDataTypeStr=int32
  nextPos_y : Inport  Port=4  OutDataTypeStr=int32
  explotion_waypoint_x : Inport  Port=5  OutDataTypeStr=int32
  explotion_waypoint_y : Inport  Port=6  OutDataTypeStr=int32
  Compare To Constant : simulink/Logic and Bit Operations/Compare To Constant  relop===  const=1  OutDataTypeStr=boolean
  Logical Operator1 : Logic  Operator=NOT  IconShape=distinctive  AllPortsSameDT=off  OutDataTypeStr=boolean
  Relational Operator : RelationalOperator  Operator===  OutDataTypeStr=boolean  RndMeth=Simplest
  Relational Operator1 : RelationalOperator  Operator===  OutDataTypeStr=boolean  RndMeth=Simplest
  and : Logic  IconShape=distinctive  AllPortsSameDT=off  OutDataTypeStr=boolean
  and1 : Logic  IconShape=distinctive  AllPortsSameDT=off  OutDataTypeStr=boolean
  or : Logic  Operator=OR  IconShape=distinctive  AllPortsSameDT=off  OutDataTypeStr=boolean
  guarantee : Outport  OutDataTypeStr=boolean
  wires:
  payload_performed/1 -> and/1
  afl2act_payloadCMD/1 -> Compare To Constant/1
  Compare To Constant/1 -> and/2
  and/1 -> Logical Operator1/1
  Logical Operator1/1 -> or/1
  or/1 -> guarantee/1
  nextPos_x/1 -> Relational Operator/1
  explotion_waypoint_x/1 -> Relational Operator/2
  nextPos_y/1 -> Relational Operator1/1
  explotion_waypoint_y/1 -> Relational Operator1/2
  Relational Operator/1 -> and1/1
  Relational Operator1/1 -> and1/2
  and1/1 -> or/2

== system benign/con_uas/c_not_taking_picture_on_arbitrary_location ==
  payload_performed : Inport  OutDataTypeStr=boolean
  afl2act_payloadCMD : Inport  Port=2  OutDataTypeStr=int32
  nextPos_x : Inport  Port=3  OutDataTypeStr=int32
  nextPos_y : Inport  Port=4  OutDataTypeStr=int32
  Compare To Constant : simulink/Logic and Bit Operations/Compare To Constant  relop===  const=0  OutDataTypeStr=boolean
  Constant : Constant  Value=0  OutDataTypeStr=int32
  Constant1 : Constant  OutDataTypeStr=int32
  Logical Operator1 : Logic  Operator=NOT  IconShape=distinctive  AllPortsSameDT=off  OutDataTypeStr=boolean
  Logical Operator2 : Logic  Operator=NOT  IconShape=distinctive  AllPortsSameDT=off  OutDataTypeStr=boolean
  Relational Operator : RelationalOperator  Operator===  OutDataTypeStr=boolean  RndMeth=Simplest
  Relational Operator1 : RelationalOperator  Operator===  OutDataTypeStr=boolean  RndMeth=Simplest
  and : Logic  IconShape=distinctive  AllPortsSameDT=off  OutDataTypeStr=boolean
  and1 : Logic  IconShape=distinctive  AllPortsSameDT=off  OutDataTypeStr=boolean
  or : Logic  Operator=OR  IconShape=distinctive  AllPortsSameDT=off  OutDataTypeStr=boolean
  guarantee : Outport  OutDataTypeStr=boolean
  wires:
  payload_performed/1 -> and/1
  afl2act_payloadCMD/1 -> Compare To Constant/1
  Compare To Constant/1 -> and/2
  and/1 -> Logical Operator1/1
  Logical Operator1/1 -> or/1
  or/1 -> guarantee/1
  nextPos_x/1 -> Relational Operator/1
  Constant/1 -> Relational Operator/2
  nextPos_y/1 -> Relational Operator1/1
  Constant1/1 -> Relational Operator1/2
  Relational Operator/1 -> and1/1
  Relational Operator1/1 -> and1/2
  and1/1 -> Logical Operator2/1
  Logical Operator2/1 -> or/2

== system benign/con_uas/d_not_releasing_weapon_on_arbitrary_location ==
  payload_performed : Inport  OutDataTypeStr=boolean
  afl2act_payloadCMD : Inport  Port=2  OutDataTypeStr=int32
  nextPos_x : Inport  Port=3  OutDataTypeStr=int32
  nextPos_y : Inport  Port=4  OutDataTypeStr=int32
  Compare To Constant : simulink/Logic and Bit Operations/Compare To Constant  relop===  const=1  OutDataTypeStr=boolean
  Constant : Constant  Value=3  OutDataTypeStr=int32
  Constant1 : Constant  OutDataTypeStr=int32
  Logical Operator1 : Logic  Operator=NOT  IconShape=distinctive  AllPortsSameDT=off  OutDataTypeStr=boolean
  Logical Operator2 : Logic  Operator=NOT  IconShape=distinctive  AllPortsSameDT=off  OutDataTypeStr=boolean
  Relational Operator : RelationalOperator  Operator===  OutDataTypeStr=boolean  RndMeth=Simplest
  Relational Operator1 : RelationalOperator  Operator===  OutDataTypeStr=boolean  RndMeth=Simplest
  and : Logic  IconShape=distinctive  AllPortsSameDT=off  OutDataTypeStr=boolean
  and1 : Logic  IconShape=distinctive  AllPortsSameDT=off  OutDataTypeStr=boolean
  or : Logic  Operator=OR  IconShape=distinctive  AllPortsSameDT=off  OutDataTypeStr=boolean
  guarantee : Outport  OutDataTypeStr=boolean
  wires:
  payload_performed/1 -> and/1
  afl2act_payloadCMD/1 -> Compare To Constant/1
  Compare To Constant/1 -> and/2
  and/1 -> Logical Operator1/1
  Logical Operator1/1 -> or/1
  or/1 -> guarantee/1
  nextPos_x/1 -> Relational Operator/1
  Constant/1 -> Relational Operator/2
  nextPos_y/1 -> Relational Operator1/1
  Constant1/1 -> Relational Operator1/2
  Relational Operator/1 -> and1/1
  Relational Operator1/1 -> and1/2
  and1/1 -> Logical Operator2/1
  Logical Operator2/1 -> or/2

== system benign/con_uas/e1_appropriate_movement_in_north ==
  nextPos_x : Inport  OutDataTypeStr=int32
  nextPos_y : Inport  Port=2  OutDataTypeStr=int32
  nextDir : Inport  Port=3  OutDataTypeStr=int32
  Add : Sum
  Logical Operator1 : Logic  Operator=NOT  IconShape=distinctive  AllPortsSameDT=off  OutDataTypeStr=boolean
  Relational Operator : RelationalOperator  Operator===  OutDataTypeStr=boolean  RndMeth=Simplest
  Relational Operator1 : RelationalOperator  Operator===  OutDataTypeStr=boolean  RndMeth=Simplest
  Relational Operator2 : RelationalOperator  Operator===  OutDataTypeStr=boolean  RndMeth=Simplest
  and : Logic  IconShape=distinctive  AllPortsSameDT=off  OutDataTypeStr=boolean
  arrow1 : CoCoSimSpecification/arrow  LustreOperatorBlock=ArrowOperator
      settings: SourceProductName=CoCoSim Specification
  one : Constant  OutDataTypeStr=int32
  or : Logic  Operator=OR  IconShape=distinctive  AllPortsSameDT=off  OutDataTypeStr=boolean
  pre_nextDir : UnitDelay  SampleTime=-1
  pre_nextPos_x : UnitDelay  SampleTime=-1
  pre_nextPos_y : UnitDelay  SampleTime=-1
  true : Constant  OutDataTypeStr=boolean
  zero : Constant  Value=0  OutDataTypeStr=int32
  guarantee : Outport  OutDataTypeStr=boolean
  wires:
  Relational Operator1/1 -> and/2
  Relational Operator/1 -> and/1
  nextPos_y/1 -> pre_nextPos_y/1, Relational Operator1/1
  nextPos_x/1 -> pre_nextPos_x/1, Relational Operator/1
  or/1 -> arrow1/2
  Logical Operator1/1 -> or/1
  true/1 -> arrow1/1
  pre_nextPos_x/1 -> Relational Operator/2
  pre_nextPos_y/1 -> Add/1
  Add/1 -> Relational Operator1/2
  one/1 -> Add/2
  nextDir/1 -> pre_nextDir/1
  pre_nextDir/1 -> Relational Operator2/1
  zero/1 -> Relational Operator2/2
  Relational Operator2/1 -> or/2
  and/1 -> Logical Operator1/1
  arrow1/1 -> guarantee/1

== system benign/con_uas/e2_appropriate_movement_in_east ==
  nextPos_x : Inport  OutDataTypeStr=int32
  nextPos_y : Inport  Port=2  OutDataTypeStr=int32
  nextDir : Inport  Port=3  OutDataTypeStr=int32
  Add1 : Sum
  Logical Operator1 : Logic  Operator=NOT  IconShape=distinctive  AllPortsSameDT=off  OutDataTypeStr=boolean
  Relational Operator : RelationalOperator  Operator===  OutDataTypeStr=boolean  RndMeth=Simplest
  Relational Operator1 : RelationalOperator  Operator===  OutDataTypeStr=boolean  RndMeth=Simplest
  Relational Operator2 : RelationalOperator  Operator===  OutDataTypeStr=boolean  RndMeth=Simplest
  and : Logic  IconShape=distinctive  AllPortsSameDT=off  OutDataTypeStr=boolean
  arrow1 : CoCoSimSpecification/arrow  LustreOperatorBlock=ArrowOperator
      settings: SourceProductName=CoCoSim Specification
  one1 : Constant  OutDataTypeStr=int32
  or : Logic  Operator=OR  IconShape=distinctive  AllPortsSameDT=off  OutDataTypeStr=boolean
  pre_nextDir : UnitDelay  SampleTime=-1
  pre_nextPos_x : UnitDelay  SampleTime=-1
  pre_nextPos_y : UnitDelay  SampleTime=-1
  true : Constant  OutDataTypeStr=boolean
  two : Constant  Value=2  OutDataTypeStr=int32
  guarantee : Outport  OutDataTypeStr=boolean
  wires:
  arrow1/1 -> guarantee/1
  and/1 -> Logical Operator1/1
  Relational Operator2/1 -> or/2
  two/1 -> Relational Operator2/2
  pre_nextDir/1 -> Relational Operator2/1
  nextDir/1 -> pre_nextDir/1
  pre_nextPos_y/1 -> Relational Operator1/2
  pre_nextPos_x/1 -> Add1/1
  true/1 -> arrow1/1
  Logical Operator1/1 -> or/1
  or/1 -> arrow1/2
  nextPos_x/1 -> Relational Operator/1, pre_nextPos_x/1
  nextPos_y/1 -> Relational Operator1/1, pre_nextPos_y/1
  Relational Operator/1 -> and/1
  Relational Operator1/1 -> and/2
  Add1/1 -> Relational Operator/2
  one1/1 -> Add1/2

== system benign/con_uas/e3_appropriate_movement_in_west ==
  nextPos_x : Inport  OutDataTypeStr=int32
  nextPos_y : Inport  Port=2  OutDataTypeStr=int32
  nextDir : Inport  Port=3  OutDataTypeStr=int32
  Add : Sum  Inputs=+-
  Logical Operator1 : Logic  Operator=NOT  IconShape=distinctive  AllPortsSameDT=off  OutDataTypeStr=boolean
  Relational Operator : RelationalOperator  Operator===  OutDataTypeStr=boolean  RndMeth=Simplest
  Relational Operator1 : RelationalOperator  Operator===  OutDataTypeStr=boolean  RndMeth=Simplest
  Relational Operator2 : RelationalOperator  Operator===  OutDataTypeStr=boolean  RndMeth=Simplest
  and : Logic  IconShape=distinctive  AllPortsSameDT=off  OutDataTypeStr=boolean
  arrow1 : CoCoSimSpecification/arrow  LustreOperatorBlock=ArrowOperator
      settings: SourceProductName=CoCoSim Specification
  one : Constant  OutDataTypeStr=int32
  or : Logic  Operator=OR  IconShape=distinctive  AllPortsSameDT=off  OutDataTypeStr=boolean
  pre_nextDir : UnitDelay  SampleTime=-1
  pre_nextPos_x : UnitDelay  SampleTime=-1
  pre_nextPos_y : UnitDelay  SampleTime=-1
  three : Constant  Value=3  OutDataTypeStr=int32
  true : Constant  OutDataTypeStr=boolean
  guarantee : Outport  OutDataTypeStr=boolean
  wires:
  Relational Operator1/1 -> and/2
  Relational Operator/1 -> and/1
  nextPos_y/1 -> pre_nextPos_y/1, Relational Operator1/1
  nextPos_x/1 -> pre_nextPos_x/1, Relational Operator/1
  or/1 -> arrow1/2
  Logical Operator1/1 -> or/1
  true/1 -> arrow1/1
  one/1 -> Add/2
  nextDir/1 -> pre_nextDir/1
  pre_nextDir/1 -> Relational Operator2/1
  three/1 -> Relational Operator2/2
  Relational Operator2/1 -> or/2
  and/1 -> Logical Operator1/1
  arrow1/1 -> guarantee/1
  Add/1 -> Relational Operator/2
  pre_nextPos_x/1 -> Add/1
  pre_nextPos_y/1 -> Relational Operator1/2

== system benign/con_uas/e4_appropriate_movement_in_north ==
  nextPos_x : Inport  OutDataTypeStr=int32
  nextPos_y : Inport  Port=2  OutDataTypeStr=int32
  nextDir : Inport  Port=3  OutDataTypeStr=int32
  Add : Sum  Inputs=+-
  Logical Operator1 : Logic  Operator=NOT  IconShape=distinctive  AllPortsSameDT=off  OutDataTypeStr=boolean
  Relational Operator : RelationalOperator  Operator===  OutDataTypeStr=boolean  RndMeth=Simplest
  Relational Operator1 : RelationalOperator  Operator===  OutDataTypeStr=boolean  RndMeth=Simplest
  Relational Operator2 : RelationalOperator  Operator===  OutDataTypeStr=boolean  RndMeth=Simplest
  and : Logic  IconShape=distinctive  AllPortsSameDT=off  OutDataTypeStr=boolean
  arrow1 : CoCoSimSpecification/arrow  LustreOperatorBlock=ArrowOperator
      settings: SourceProductName=CoCoSim Specification
  one : Constant  OutDataTypeStr=int32
  one1 : Constant  OutDataTypeStr=int32
  or : Logic  Operator=OR  IconShape=distinctive  AllPortsSameDT=off  OutDataTypeStr=boolean
  pre_nextDir : UnitDelay  SampleTime=-1
  pre_nextPos_x : UnitDelay  SampleTime=-1
  pre_nextPos_y : UnitDelay  SampleTime=-1
  true : Constant  OutDataTypeStr=boolean
  guarantee : Outport  OutDataTypeStr=boolean
  wires:
  arrow1/1 -> guarantee/1
  and/1 -> Logical Operator1/1
  Relational Operator2/1 -> or/2
  one1/1 -> Relational Operator2/2
  pre_nextDir/1 -> Relational Operator2/1
  nextDir/1 -> pre_nextDir/1
  one/1 -> Add/2
  Add/1 -> Relational Operator1/2
  pre_nextPos_y/1 -> Add/1
  pre_nextPos_x/1 -> Relational Operator/2
  true/1 -> arrow1/1
  Logical Operator1/1 -> or/1
  or/1 -> arrow1/2
  nextPos_x/1 -> Relational Operator/1, pre_nextPos_x/1
  nextPos_y/1 -> Relational Operator1/1, pre_nextPos_y/1
  Relational Operator/1 -> and/1
  Relational Operator1/1 -> and/2

== system benign/uas/RC_receiver ==
  rcv_MIE1 : Inport  OutDataTypeStr=int32
  rcv_MIE2 : Inport  Port=2  OutDataTypeStr=int32
  rcv_MIE3 : Inport  Port=3  OutDataTypeStr=int32
  rcv_MIE4 : Inport  Port=4  OutDataTypeStr=int32
  true : Constant  OutDataTypeStr=boolean
  normal : Outport  OutDataTypeStr=boolean
  MIE1 : Outport  Port=2  OutDataTypeStr=int32
  MIE2 : Outport  Port=3  OutDataTypeStr=int32
  MIE3 : Outport  Port=4  OutDataTypeStr=int32
  MIE4 : Outport  Port=5  OutDataTypeStr=int32
  wires:
  rcv_MIE4/1 -> MIE4/1
  rcv_MIE3/1 -> MIE3/1
  rcv_MIE2/1 -> MIE2/1
  rcv_MIE1/1 -> MIE1/1
  true/1 -> normal/1

== system benign/uas/RC_receiver_health_check ==
  normal : Inport  OutDataTypeStr=boolean
  Relational Operator : RelationalOperator  Operator=<=  OutDataTypeStr=boolean  RndMeth=Simplest
  Switch : Switch  Criteria=u2 > Threshold
  duration : Subsystem
  one : Constant  OutDataTypeStr=int32
  tolerance_level : Constant  OutDataTypeStr=int32
  zero : Constant  Value=0  OutDataTypeStr=int32
  ATE6 : Outport  OutDataTypeStr=int32
  wires:
  normal/1 -> duration/1(p)
  duration/1(r) -> Relational Operator/1
  tolerance_level/1 -> Relational Operator/2
  Relational Operator/1 -> Switch/2
  one/1 -> Switch/1
  zero/1 -> Switch/3
  Switch/1 -> ATE6/1

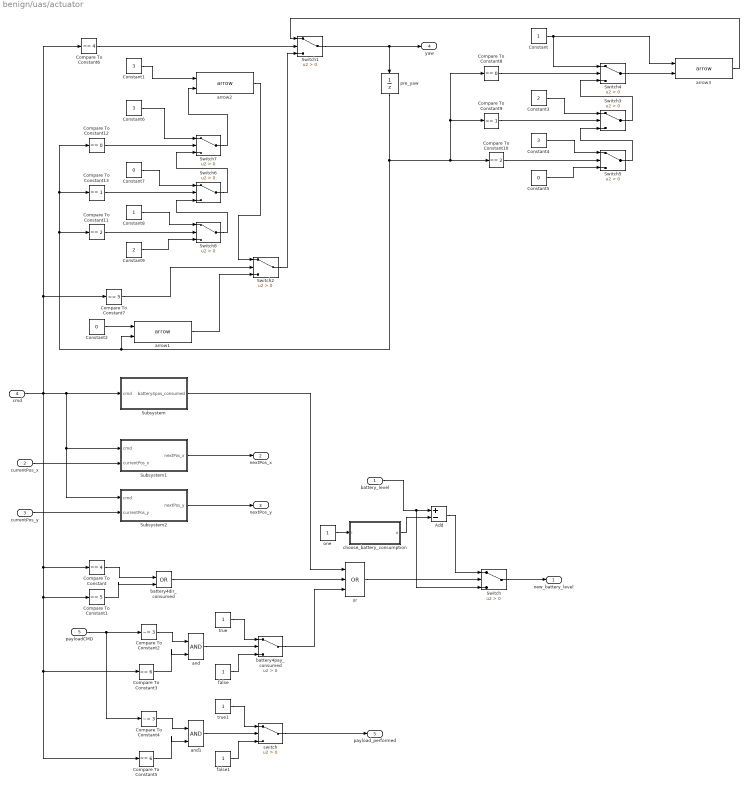
== system benign/uas/actuator ==
  battery_level : Inport  OutDataTypeStr=int32
  currentPos_x : Inport  Port=2  OutDataTypeStr=int32
  currentPos_y : Inport  Port=3  OutDataTypeStr=int32
  cmd : Inport  Port=4  OutDataTypeStr=int32
  payloadCMD : Inport  Port=5  OutDataTypeStr=int32
  Add : Sum  Inputs=+-
  Compare To Constant : simulink/Logic and Bit Operations/Compare To Constant  relop===  const=4  OutDataTypeStr=boolean
  Compare To Constant1 : simulink/Logic and Bit Operations/Compare To Constant  relop===  const=5  OutDataTypeStr=boolean
  Compare To Constant10 : simulink/Logic and Bit Operations/Compare To Constant  relop===  const=2  OutDataTypeStr=boolean
  Compare To Constant11 : simulink/Logic and Bit Operations/Compare To Constant  relop===  const=2  OutDataTypeStr=boolean
  Compare To Constant12 : simulink/Logic and Bit Operations/Compare To Constant  relop===  const=0  OutDataTypeStr=boolean
  Compare To Constant13 : simulink/Logic and Bit Operations/Compare To Constant  relop===  const=1  OutDataTypeStr=boolean
  Compare To Constant2 : simulink/Logic and Bit Operations/Compare To Constant  relop=~=  const=3  OutDataTypeStr=boolean
  Compare To Constant3 : simulink/Logic and Bit Operations/Compare To Constant  relop===  const=6  OutDataTypeStr=boolean
  Compare To Constant4 : simulink/Logic and Bit Operations/Compare To Constant  relop=~=  const=3  OutDataTypeStr=boolean
  Compare To Constant5 : simulink/Logic and Bit Operations/Compare To Constant  relop===  const=6  OutDataTypeStr=boolean
  Compare To Constant6 : simulink/Logic and Bit Operations/Compare To Constant  relop===  const=4  OutDataTypeStr=boolean
  Compare To Constant7 : simulink/Logic and Bit Operations/Compare To Constant  relop===  const=5  OutDataTypeStr=boolean
  Compare To Constant8 : simulink/Logic and Bit Operations/Compare To Constant  relop===  const=0  OutDataTypeStr=boolean
  Compare To Constant9 : simulink/Logic and Bit Operations/Compare To Constant  relop===  const=1  OutDataTypeStr=boolean
  Constant : Constant  OutDataTypeStr=int32
  Constant1 : Constant  Value=3  OutDataTypeStr=int32
  Constant2 : Constant  Value=0  OutDataTypeStr=int32
  Constant3 : Constant  Value=2  OutDataTypeStr=int32
  Constant4 : Constant  Value=3  OutDataTypeStr=int32
  Constant5 : Constant  Value=0  OutDataTypeStr=int32
  Constant6 : Constant  Value=3  OutDataTypeStr=int32
  Constant7 : Constant  Value=0  OutDataTypeStr=int32
  Constant8 : Constant  OutDataTypeStr=int32
  Constant9 : Constant  Value=2  OutDataTypeStr=int32
  Subsystem : Subsystem
  Subsystem1 : Subsystem
  Subsystem2 : Subsystem
  Switch{,1..8} (9 alike) : Switch  Criteria=u2 > Threshold
  and : Logic  IconShape=distinctive  AllPortsSameDT=off  OutDataTypeStr=boolean
  and1 : Logic  IconShape=distinctive  AllPortsSameDT=off  OutDataTypeStr=boolean
  arrow1 : CoCoSimSpecification/arrow  LustreOperatorBlock=ArrowOperator
      settings: SourceProductName=CoCoSim Specification
  arrow2 : CoCoSimSpecification/arrow  LustreOperatorBlock=ArrowOperator
      settings: SourceProductName=CoCoSim Specification
  arrow3 : CoCoSimSpecification/arrow  LustreOperatorBlock=ArrowOperator
      settings: SourceProductName=CoCoSim Specification
  battery4dir_consumed : Logic  Operator=OR  IconShape=distinctive  AllPortsSameDT=off  OutDataTypeStr=boolean
  battery4pay_consumed : Switch  Criteria=u2 > Threshold
  choose_battery_consumption : Subsystem
  false : Constant  OutDataTypeStr=boolean
  false1 : Constant  OutDataTypeStr=boolean
  one : Constant  OutDataTypeStr=int32
  or : Logic  Operator=OR  Inputs=3  IconShape=distinctive  AllPortsSameDT=off  OutDataTypeStr=boolean
  pre_yaw : UnitDelay  SampleTime=-1
  switch : Switch  Criteria=u2 > Threshold
  true : Constant  OutDataTypeStr=boolean
  true1 : Constant  OutDataTypeStr=boolean
  new_battery_level : Outport  OutDataTypeStr=int32
  nextPos_x : Outport  Port=2  OutDataTypeStr=int32
  nextPos_y : Outport  Port=3  OutDataTypeStr=int32
  yaw : Outport  Port=4  OutDataTypeStr=int32
  payload_performed : Outport  Port=5  OutDataTypeStr=boolean
  wires:
  Subsystem1/1(nextPos_x) -> nextPos_x/1
  currentPos_x/1 -> Subsystem1/2(currentPos_x)
  Subsystem2/1(nextPos_y) -> nextPos_y/1
  currentPos_y/1 -> Subsystem2/2(currentPos_y)
  Compare To Constant/1 -> battery4dir_consumed/1
  Compare To Constant1/1 -> battery4dir_consumed/2
  battery4dir_consumed/1 -> or/2
  Subsystem/1(battery4pos_consumed) -> or/1
  battery_level/1 -> Switch/3, Add/1
  choose_battery_consumption/1(o) -> Add/2
  or/1 -> Switch/2
  Add/1 -> Switch/1
  one/1 -> choose_battery_consumption/1(i)
  Switch/1 -> new_battery_level/1
  Compare To Constant2/1 -> and/1
  Compare To Constant3/1 -> and/2
  and/1 -> battery4pay_consumed/2
  true/1 -> battery4pay_consumed/1
  false/1 -> battery4pay_consumed/3
  battery4pay_consumed/1 -> or/3
  switch/1 -> payload_performed/1
  true1/1 -> switch/1
  Compare To Constant5/1 -> and1/2
  false1/1 -> switch/3
  Compare To Constant4/1 -> and1/1
  cmd/1 -> Compare To Constant6/1, Compare To Constant7/1, Compare To Constant1/1, Compare To Constant5/1, Compare To Constant3/1, Compare To Constant/1, Subsystem2/1(cmd), Subsystem1/1(cmd), Subsystem/1(cmd)
  payloadCMD/1 -> Compare To Constant4/1, Compare To Constant2/1
  and1/1 -> switch/2
  Compare To Constant6/1 -> Switch1/2
  Switch1/1 -> pre_yaw/1, yaw/1
  Switch2/1 -> Switch1/3
  Constant/1 -> Switch4/1, arrow3/1
  Constant1/1 -> arrow2/1
  Constant2/1 -> arrow1/1
  arrow3/1 -> Switch1/1
  arrow2/1 -> Switch2/1
  Compare To Constant7/1 -> Switch2/2
  arrow1/1 -> Switch2/3
  pre_yaw/1 -> Compare To Constant10/1, Compare To Constant9/1, Compare To Constant8/1, Compare To Constant13/1, Compare To Constant12/1, Compare To Constant11/1, arrow1/2
  Compare To Constant8/1 -> Switch4/2
  Switch4/1 -> arrow3/2
  Switch3/1 -> Switch4/3
  Compare To Constant9/1 -> Switch3/2
  Constant3/1 -> Switch3/1
  Compare To Constant10/1 -> Switch5/2
  Constant4/1 -> Switch5/1
  Constant5/1 -> Switch5/3
  Switch5/1 -> Switch3/3
  Constant6/1 -> Switch7/1
  Constant7/1 -> Switch6/1
  Compare To Constant11/1 -> Switch8/2
  Switch6/1 -> Switch7/3
  Compare To Constant13/1 -> Switch6/2
  Constant8/1 -> Switch8/1
  Switch8/1 -> Switch6/3
  Constant9/1 -> Switch8/3
  Switch7/1 -> arrow2/2
  Compare To Constant12/1 -> Switch7/2
